simulink model "eVTOL_System"  (R2024b)
settings: Solver=FixedStepAuto  StartTime=0.0  StopTime=inf  RelTol=1e-3
undefined symbols (not defined in the file): airspeed, Battery, BCE12, BCE_Set_init, BMS_Controller_State, C, Cell10_P, Cell11_P, Cell12_P, Cell13_P, Cell14_P, Cell15_P, Cell16_P, Cell17_P, Cell18_P, Cell19_P, Cell1_N, Cell1_P, Cell20_P, Cell21_P, Cell22_P, Cell23_P, Cell24_P, Cell2_P, Cell3_P, Cell4_P, Cell5_P, Cell6_P, Cell7_P, Cell8_P, Cell9_P, Charging_State, CityMission, control, controlParams, ControlSampleTime, CriticalTiltAngle, currentFactor, CV_Gain, ddx, ddy, ddz, Device_01, Device_02, DiscIntNeverNeededParam, dx, dy, dz, Earth, env, F, F28379D_ADC_MaxCount, F28379D_ADC_Vmax, FixedWingMission, flightState, Foc_Ki_IxTcpu, Foc_Ki_S, Foc_Kp_I, Foc_Kp_S, fractalcoef ... (+68)
libraries: fl_lib x1115, nesl_utility x617, slrealtimeethercatlib x217, simulink x130, canmsglib x101, speedgoatlib_IO611_obsolete x91, slpidlib x49, mcbcontrolslib x44, slrealtimeutilitieslib x35, speedgoatlib_hdlCoder_IO3xx x31, dspstat3 x24, mcbpositiondecoderlib x12
(part 30 of 31)

== system eVTOL_System/Motor Drive/Controller2/Controller_MIL/F28379D Firmware/Controller Algorithm/FOC/Current Control/Control_System/Closed Loop Control/Subsystem/Current_Controllers/PI_Controller_Iq ==
  I_ref : Inport
  I_fb : Inport  Port=2
  EnablePWM : Inport  Port=3
  Kp_i : Inport  Port=4
  Ki_ixTcpu : Inport  Port=5
  Discrete PI Controller with anti-windup & reset : slpidlib/PID Controller  Controller=PI  Form=Parallel  TimeDomain=Discrete-time  UseExternalTs=off  SampleTime=-1  IntegratorMethod=Forward Euler  FilterMethod=Forward Euler  ControllerParametersSource=external  P=1  I=1  UseKiTs=on  D=0  UseExternalDerivativeSource=off  N=100  UseFilter=on  TunerSelectOption=Transfer Function Based (PID Tuner App)  InitialConditionSource=external  InitialConditionForIntegrator=0  InitialConditionForFilter=0  DifferentiatorICPrevScaledInput=0  ExternalReset=level  TrackingMode=off  Kt=1  LimitOutput=on  SatLimitsSource=internal  UpperSaturationLimit=1  LowerSaturationLimit=-1  LinearizeAsGain=on  AntiWindupMode=clamping  Kb=1  LimitIntegrator=off  UpperIntegratorSaturationLimit=inf  LowerIntegratorSaturationLimit=-inf  RndMeth=Simplest  POutMin=[]  POutMax=[]  IOutMin=[]  IOutMax=[]  DOutMin=[]  DOutMax=[]  NOutMin=[]  NOutMax=[]  SumOutMin=[]  SumOutMax=[]  SaturationOutDataTypeStr=Inherit: Inherit via back propagation  SaturationOutMin=[]  SaturationOutMax=[]  PParamMin=[]  PParamMax=[]  IParamMin=[]  IParamMax=[]  DParamMin=[]  DParamMax=[]  NParamMin=[]  NParamMax=[]  KbParamMin=[]  KbParamMax=[]  KtParamMin=[]  KtParamMax=[]  KbOutMin=[]  KbOutMax=[]  KtOutMin=[]  KtOutMax=[]  IntegratorOutMin=[]  IntegratorOutMax=[]  FilterOutMin=[]  FilterOutMax=[]  SumI1OutMin=[]  SumI1OutMax=[]  SumI2OutMin=[]  SumI2OutMax=[]  SumI3OutMin=[]  SumI3OutMax=[]  SumI4OutMin=[]  SumI4OutMax=[]  SumDOutMin=[]  SumDOutMax=[]  DifferentiatorOutMin=[]  DifferentiatorOutMax=[]  FilterDiffOutCoefMin=[]  FilterDiffOutCoefMax=[]  ReciprocalOutMin=[]  ReciprocalOutMax=[]  SumDenOutMin=[]  SumDenOutMax=[]  SumNumOutMin=[]  SumNumOutMax=[]  DivideOutMin=[]  DivideOutMax=[]  UdiffTsProdOutMin=[]  UdiffTsProdOutMax=[]  NTsProdOutMin=[]  NTsProdOutMax=[]  UintegralTsProdOutMin=[]  UintegralTsProdOutMax=[]  UngainTsProdOutMin=[]  UngainTsProdOutMax=[]  ClampingZeroOutDataTypeStr=Inherit: Inherit via back propagation  ClampingZeroOutMin=[]  ClampingZeroOutMax=[]  FilterDenConstantOutDataTypeStr=Inherit: Inherit via back propagation  FilterDenConstantOutMin=[]  FilterDenConstantOutMax=[]  PCopyOutDataTypeStr=Inherit: Inherit via back propagation  PCopyOutMin=[]  PCopyOutMax=[]  NCopyOutDataTypeStr=Inherit: Inherit via back propagation  NCopyOutMin=[]  NCopyOutMax=[]  IntegratorContinuousStateAttributes=''  IntegratorStateMustResolveToSignalObject=off  IntegratorRTWStateStorageClass=Auto  FilterContinuousStateAttributes=''  FilterStateMustResolveToSignalObject=off  FilterRTWStateStorageClass=Auto  ParallelPVariant=ExternalParameters  IdealPVariant=Disabled  IVariant=ExternalParameters  DVariant=Disabled  IntegratorVariant=Discrete  SatVariant=Enabled  AWVariant=DiscClampingParallel  PCopyVariant=Disabled  TRVariant=Disabled  FdbkBlocksVariant=Forward  IdealPFdbkVariant=Disabled  SatFdbkVariant=Disabled  DerivativeFilterVariant=Disabled  NVariant=Disabled  NCopyVariant=Disabled_SignalSpec  FilterICVariant=Disabled  IntegratorICVariant=ExternalICs  ExternalResetVariant=ExternalReset  TRSumVariant=Passthrough  SumFdbkVariant=Disabled  SumVariant=Sum_PI  TsampFilterVariant=InternalTs  TsampNgainVariant=Passthrough  TsampIntegralVariant=Disabled_SignalSpec  ExternalSaturationOutDataTypeStr=Inherit: Same as second input  DerivativeSourceVariant=Disabled  PreIntVariant=InternalPreInt
  Kp1 : Constant  Value=0  OutDataTypeStr=single  SampleTime=-1
  Logical Operator : Logic  Operator=NOT  IconShape=distinctive  AllPortsSameDT=off  OutDataTypeStr=boolean
  Sum : Sum  Inputs=|+-  OutDataTypeStr=Inherit: Same as first input
  V_ref : Outport  VectorParamsAs1DForOutWhenUnconnected=off
  wires:
  Discrete PI Controller with anti-windup & reset/1 -> V_ref/1
  I_fb/1 -> Sum/2
  I_ref/1 -> Sum/1
  Sum/1 -> Discrete PI Controller with anti-windup & reset/1
  Logical Operator/1 -> Discrete PI Controller with anti-windup & reset/4
  Kp1/1 -> Discrete PI Controller with anti-windup & reset/5
  EnablePWM/1 -> Logical Operator/1
  Kp_i/1 -> Discrete PI Controller with anti-windup & reset/2
  Ki_ixTcpu/1 -> Discrete PI Controller with anti-windup & reset/3

== system eVTOL_System/Motor Drive/Controller3/Controller_MIL/F28379D Firmware/Controller Algorithm/FOC/Current Control/Control_System/Closed Loop Control/Subsystem/Current_Controllers/PI_Controller_Id ==
  I_ref : Inport
  I_fb : Inport  Port=2
  EnablePWM : Inport  Port=3
  Kp_i : Inport  Port=4
  Ki_ixTcpu : Inport  Port=5
  Discrete PI Controller with anti-windup & reset : slpidlib/PID Controller  Controller=PI  Form=Parallel  TimeDomain=Discrete-time  UseExternalTs=off  SampleTime=-1  IntegratorMethod=Forward Euler  FilterMethod=Forward Euler  ControllerParametersSource=external  P=1  I=1  UseKiTs=on  D=0  UseExternalDerivativeSource=off  N=100  UseFilter=on  TunerSelectOption=Transfer Function Based (PID Tuner App)  InitialConditionSource=external  InitialConditionForIntegrator=0  InitialConditionForFilter=0  DifferentiatorICPrevScaledInput=0  ExternalReset=level  TrackingMode=off  Kt=1  LimitOutput=on  SatLimitsSource=internal  UpperSaturationLimit=1  LowerSaturationLimit=-1  LinearizeAsGain=on  AntiWindupMode=clamping  Kb=1  LimitIntegrator=off  UpperIntegratorSaturationLimit=inf  LowerIntegratorSaturationLimit=-inf  RndMeth=Simplest  POutMin=[]  POutMax=[]  IOutMin=[]  IOutMax=[]  DOutMin=[]  DOutMax=[]  NOutMin=[]  NOutMax=[]  SumOutMin=[]  SumOutMax=[]  SaturationOutDataTypeStr=Inherit: Inherit via back propagation  SaturationOutMin=[]  SaturationOutMax=[]  PParamMin=[]  PParamMax=[]  IParamMin=[]  IParamMax=[]  DParamMin=[]  DParamMax=[]  NParamMin=[]  NParamMax=[]  KbParamMin=[]  KbParamMax=[]  KtParamMin=[]  KtParamMax=[]  KbOutMin=[]  KbOutMax=[]  KtOutMin=[]  KtOutMax=[]  IntegratorOutMin=[]  IntegratorOutMax=[]  FilterOutMin=[]  FilterOutMax=[]  SumI1OutMin=[]  SumI1OutMax=[]  SumI2OutMin=[]  SumI2OutMax=[]  SumI3OutMin=[]  SumI3OutMax=[]  SumI4OutMin=[]  SumI4OutMax=[]  SumDOutMin=[]  SumDOutMax=[]  DifferentiatorOutMin=[]  DifferentiatorOutMax=[]  FilterDiffOutCoefMin=[]  FilterDiffOutCoefMax=[]  ReciprocalOutMin=[]  ReciprocalOutMax=[]  SumDenOutMin=[]  SumDenOutMax=[]  SumNumOutMin=[]  SumNumOutMax=[]  DivideOutMin=[]  DivideOutMax=[]  UdiffTsProdOutMin=[]  UdiffTsProdOutMax=[]  NTsProdOutMin=[]  NTsProdOutMax=[]  UintegralTsProdOutMin=[]  UintegralTsProdOutMax=[]  UngainTsProdOutMin=[]  UngainTsProdOutMax=[]  ClampingZeroOutDataTypeStr=Inherit: Inherit via back propagation  ClampingZeroOutMin=[]  ClampingZeroOutMax=[]  FilterDenConstantOutDataTypeStr=Inherit: Inherit via back propagation  FilterDenConstantOutMin=[]  FilterDenConstantOutMax=[]  PCopyOutDataTypeStr=Inherit: Inherit via back propagation  PCopyOutMin=[]  PCopyOutMax=[]  NCopyOutDataTypeStr=Inherit: Inherit via back propagation  NCopyOutMin=[]  NCopyOutMax=[]  IntegratorContinuousStateAttributes=''  IntegratorStateMustResolveToSignalObject=off  IntegratorRTWStateStorageClass=Auto  FilterContinuousStateAttributes=''  FilterStateMustResolveToSignalObject=off  FilterRTWStateStorageClass=Auto  ParallelPVariant=ExternalParameters  IdealPVariant=Disabled  IVariant=ExternalParameters  DVariant=Disabled  IntegratorVariant=Discrete  SatVariant=Enabled  AWVariant=DiscClampingParallel  PCopyVariant=Disabled  TRVariant=Disabled  FdbkBlocksVariant=Forward  IdealPFdbkVariant=Disabled  SatFdbkVariant=Disabled  DerivativeFilterVariant=Disabled  NVariant=Disabled  NCopyVariant=Disabled_SignalSpec  FilterICVariant=Disabled  IntegratorICVariant=ExternalICs  ExternalResetVariant=ExternalReset  TRSumVariant=Passthrough  SumFdbkVariant=Disabled  SumVariant=Sum_PI  TsampFilterVariant=InternalTs  TsampNgainVariant=Passthrough  TsampIntegralVariant=Disabled_SignalSpec  ExternalSaturationOutDataTypeStr=Inherit: Same as second input  DerivativeSourceVariant=Disabled  PreIntVariant=InternalPreInt
  Ki1 : Constant  Value=0  OutDataTypeStr=single  SampleTime=-1
  Logical Operator : Logic  Operator=NOT  IconShape=distinctive  AllPortsSameDT=off  OutDataTypeStr=boolean
  Sum : Sum  Inputs=|+-  OutDataTypeStr=Inherit: Same as first input
  V_ref : Outport  VectorParamsAs1DForOutWhenUnconnected=off
  wires:
  I_ref/1 -> Sum/1
  I_fb/1 -> Sum/2
  Discrete PI Controller with anti-windup & reset/1 -> V_ref/1
  Sum/1 -> Discrete PI Controller with anti-windup & reset/1
  Logical Operator/1 -> Discrete PI Controller with anti-windup & reset/4
  Ki1/1 -> Discrete PI Controller with anti-windup & reset/5
  EnablePWM/1 -> Logical Operator/1
  Kp_i/1 -> Discrete PI Controller with anti-windup & reset/2
  Ki_ixTcpu/1 -> Discrete PI Controller with anti-windup & reset/3

== system eVTOL_System/Motor Drive/Controller3/Controller_MIL/F28379D Firmware/Controller Algorithm/FOC/Current Control/Control_System/Closed Loop Control/Subsystem/Current_Controllers/PI_Controller_Iq ==
  I_ref : Inport
  I_fb : Inport  Port=2
  EnablePWM : Inport  Port=3
  Kp_i : Inport  Port=4
  Ki_ixTcpu : Inport  Port=5
  Discrete PI Controller with anti-windup & reset : slpidlib/PID Controller  Controller=PI  Form=Parallel  TimeDomain=Discrete-time  UseExternalTs=off  SampleTime=-1  IntegratorMethod=Forward Euler  FilterMethod=Forward Euler  ControllerParametersSource=external  P=1  I=1  UseKiTs=on  D=0  UseExternalDerivativeSource=off  N=100  UseFilter=on  TunerSelectOption=Transfer Function Based (PID Tuner App)  InitialConditionSource=external  InitialConditionForIntegrator=0  InitialConditionForFilter=0  DifferentiatorICPrevScaledInput=0  ExternalReset=level  TrackingMode=off  Kt=1  LimitOutput=on  SatLimitsSource=internal  UpperSaturationLimit=1  LowerSaturationLimit=-1  LinearizeAsGain=on  AntiWindupMode=clamping  Kb=1  LimitIntegrator=off  UpperIntegratorSaturationLimit=inf  LowerIntegratorSaturationLimit=-inf  RndMeth=Simplest  POutMin=[]  POutMax=[]  IOutMin=[]  IOutMax=[]  DOutMin=[]  DOutMax=[]  NOutMin=[]  NOutMax=[]  SumOutMin=[]  SumOutMax=[]  SaturationOutDataTypeStr=Inherit: Inherit via back propagation  SaturationOutMin=[]  SaturationOutMax=[]  PParamMin=[]  PParamMax=[]  IParamMin=[]  IParamMax=[]  DParamMin=[]  DParamMax=[]  NParamMin=[]  NParamMax=[]  KbParamMin=[]  KbParamMax=[]  KtParamMin=[]  KtParamMax=[]  KbOutMin=[]  KbOutMax=[]  KtOutMin=[]  KtOutMax=[]  IntegratorOutMin=[]  IntegratorOutMax=[]  FilterOutMin=[]  FilterOutMax=[]  SumI1OutMin=[]  SumI1OutMax=[]  SumI2OutMin=[]  SumI2OutMax=[]  SumI3OutMin=[]  SumI3OutMax=[]  SumI4OutMin=[]  SumI4OutMax=[]  SumDOutMin=[]  SumDOutMax=[]  DifferentiatorOutMin=[]  DifferentiatorOutMax=[]  FilterDiffOutCoefMin=[]  FilterDiffOutCoefMax=[]  ReciprocalOutMin=[]  ReciprocalOutMax=[]  SumDenOutMin=[]  SumDenOutMax=[]  SumNumOutMin=[]  SumNumOutMax=[]  DivideOutMin=[]  DivideOutMax=[]  UdiffTsProdOutMin=[]  UdiffTsProdOutMax=[]  NTsProdOutMin=[]  NTsProdOutMax=[]  UintegralTsProdOutMin=[]  UintegralTsProdOutMax=[]  UngainTsProdOutMin=[]  UngainTsProdOutMax=[]  ClampingZeroOutDataTypeStr=Inherit: Inherit via back propagation  ClampingZeroOutMin=[]  ClampingZeroOutMax=[]  FilterDenConstantOutDataTypeStr=Inherit: Inherit via back propagation  FilterDenConstantOutMin=[]  FilterDenConstantOutMax=[]  PCopyOutDataTypeStr=Inherit: Inherit via back propagation  PCopyOutMin=[]  PCopyOutMax=[]  NCopyOutDataTypeStr=Inherit: Inherit via back propagation  NCopyOutMin=[]  NCopyOutMax=[]  IntegratorContinuousStateAttributes=''  IntegratorStateMustResolveToSignalObject=off  IntegratorRTWStateStorageClass=Auto  FilterContinuousStateAttributes=''  FilterStateMustResolveToSignalObject=off  FilterRTWStateStorageClass=Auto  ParallelPVariant=ExternalParameters  IdealPVariant=Disabled  IVariant=ExternalParameters  DVariant=Disabled  IntegratorVariant=Discrete  SatVariant=Enabled  AWVariant=DiscClampingParallel  PCopyVariant=Disabled  TRVariant=Disabled  FdbkBlocksVariant=Forward  IdealPFdbkVariant=Disabled  SatFdbkVariant=Disabled  DerivativeFilterVariant=Disabled  NVariant=Disabled  NCopyVariant=Disabled_SignalSpec  FilterICVariant=Disabled  IntegratorICVariant=ExternalICs  ExternalResetVariant=ExternalReset  TRSumVariant=Passthrough  SumFdbkVariant=Disabled  SumVariant=Sum_PI  TsampFilterVariant=InternalTs  TsampNgainVariant=Passthrough  TsampIntegralVariant=Disabled_SignalSpec  ExternalSaturationOutDataTypeStr=Inherit: Same as second input  DerivativeSourceVariant=Disabled  PreIntVariant=InternalPreInt
  Kp1 : Constant  Value=0  OutDataTypeStr=single  SampleTime=-1
  Logical Operator : Logic  Operator=NOT  IconShape=distinctive  AllPortsSameDT=off  OutDataTypeStr=boolean
  Sum : Sum  Inputs=|+-  OutDataTypeStr=Inherit: Same as first input
  V_ref : Outport  VectorParamsAs1DForOutWhenUnconnected=off
  wires:
  Discrete PI Controller with anti-windup & reset/1 -> V_ref/1
  I_fb/1 -> Sum/2
  I_ref/1 -> Sum/1
  Sum/1 -> Discrete PI Controller with anti-windup & reset/1
  Logical Operator/1 -> Discrete PI Controller with anti-windup & reset/4
  Kp1/1 -> Discrete PI Controller with anti-windup & reset/5
  EnablePWM/1 -> Logical Operator/1
  Kp_i/1 -> Discrete PI Controller with anti-windup & reset/2
  Ki_ixTcpu/1 -> Discrete PI Controller with anti-windup & reset/3

== matlab function eVTOL_System/Flight Controller/Autopilot/Fixed Wing Controller/Fixed Wing Controller Simulation/Attitude Controller/Pitch Roll Controller/Turn Coordinator/MATLAB Function ==
  data: rollSP input; rSP output; pitchSP input; airSpeed input
function rSP = fcn(rollSP, pitchSP, airSpeed)
    yawRateSP = tan(rollSP)*9.81/airSpeed;
    rSP = yawRateSP*cos(pitchSP)*cos(rollSP);
end

== stateflow chart eVTOL_System/Flight Controller/Guidance Test Bench/ControlType/Guidance Testbench/Guidance Logic/Guidance Stateflow/Guidance Mode Selector ==
  settings: updateMethod=DISCRETE  sampleTime=UAVSampleTime*4
  state GuidanceLogic
    state FIXED_WING_WAYPOINT
      en:
      controlMode.airspeedAltitude = 1;
      controlMode.attitude = 1;
      controlMode.lateralGuidance = 1;
      state WAYPOINT
    state FIXED_WING_ENTRY
      state Stabilize
        en:
        FlightMode=flightState.FixedWing;
        controlMode.attitude = 1;
        controlMode.airspeedAltitude = 0;
        controlMode.lateralGuidance = 0;
        %Transition once done.
        FixedWingSP.yaw = 0;
        FixedWingSP.pitch = 0;
        FixedWingSP.roll = 0;
        FixedWingSP.airspeed=14;
        Status= uint8(0);
      state FIXEDWINGFLIGHT
        en:
        % Control mode
        controlMode.airspeedAltitude = 1;
        controlMode.attitude = 1;
        controlMode.lateralGuidance = 1;
        % Setpoint init
        aacSP.L1 = 25;
        aacSP.airspeed = 14;
        aacSP.altitude = 0;
        aacSP.course=0;
      (default) -> Stabilize
      Stabilize -> FIXEDWINGFLIGHT : after(3,sec)
    state Start
      en:
      %Set Flight mode to hover
      FlightMode=PresetMode;
      %Set default settings
      % Control mode
      controlMode.airspeedAltitude = 0;
      controlMode.attitude = 0;
      controlMode.lateralGuidance = 0;
      controlMode.TransitionCondition = 0;
      % Setpoint init
      FixedWingSP.yaw = 0;
      FixedWingSP.pitch = 0;
      FixedWingSP.roll = 0;
      FixedWingSP.airspeed=14;
      aacSP.L1 = 25;
      aacSP.airspeed = 14;
      aacSP.altitude = 0;
      aacSP.course=0;
      InnerLoopCmds.YawCmd=0;
    state FIXED_WING_ORBIT
      en:
      controlMode.airspeedAltitude = 1;
      controlMode.attitude = 1;
      controlMode.lateralGuidance = 1;
      state ORBIT
    state HOVER_ENTRY
      en:
      FlightMode=flightState.Hover;
      controlMode.inTransition=0;
    state Takeoff
    state WP
    state Orbit
    state PreTransition
      en:
      FlightMode=flightState.FixedWing;
      controlMode.airspeedAltitude = 1;
      controlMode.attitude = 1;
      controlMode.lateralGuidance = 1;
      % Setpoint init
      aacSP.L1 = 25;
      aacSP.airspeed = 14;
      aacSP.altitude = altitudeHold;
      aacSP.course=courseHold;
    state BackTransition
      state BackTransition
    state ForwardTransition
    state FWCOMPLETE
      Status=uint8(1);
      controlMode.TransitionCondition=uint8(1);
    note: [(mode==4)]
    state Land
      state Descend
      state WingsLevel
      state ToLand
      (default) -> ToLand
      WingsLevel -> Descend : [isLevel(States)]
      ToLand -> WingsLevel : [(norm(Pose(1:2)-ToWP.position(1:2)) <= 5)]
    (default) -> Start
    Start -> (junction 5)
    FIXEDWINGFLIGHT -> WAYPOINT [order 2] : [(mode==2)]
        | {Status=uint8(0);}
    FIXEDWINGFLIGHT -> ORBIT [order 1] : [(mode==3)]
        | {Status= uint8(0);}
    (junction 262) -> FIXED_WING_ENTRY
    (junction 5) -> FIXED_WING_ORBIT [order 6] : [(mode==3)&&(FlightMode==flightState.FixedWing)]
        | {Status=uint8(0);}
    (junction 5) -> (junction 262) [order 3] : [(FlightMode==flightState.Transition)]
        | {controlMode.inTransition=0;}
    (junction 255) -> HOVER_ENTRY
    (junction 5) -> (junction 255) [order 4] : [(FlightMode==flightState.BackTransition)]
        | {controlMode.inTransition=0;}
    HOVER_ENTRY -> (junction 12)
    (junction 257) -> FIXED_WING_WAYPOINT
    Takeoff -> WP : [Pose(3) <= ToWP.position(3)]{Status = uint8(1);}
    GuidanceLogic -> (junction 5) : [(hasChanged(mode))]
    (junction 5) -> Takeoff [order 5] : [(mode == 1)&&(FlightMode==flightState.Hover)]
        | {controlMode.inTransition=0;}
    (junction 5) -> (junction 257) [order 2] : [(mode==2)&&(FlightMode==flightState.FixedWing)]
        | {Status=uint8(0);}
    (junction 5) -> (junction 260) [order 1] : [(mode==6)&&(FlightMode==flightState.FixedWing)]
        | {courseHold=States.course;
        | altitudeHold=-States.Xe(3); }
    (junction 5) -> (junction 12) [order 7] : [FlightMode==flightState.Hover]
        | {controlMode.inTransition=0;}
    (junction 260) -> PreTransition
    (junction 12) -> WP [order 1] : [(mode==2)]
    (junction 12) -> (junction 17) [order 2]
    (junction 17) -> Orbit [order 1] : [(mode==3)]
    (junction 17) -> (junction 22) [order 2]
    PreTransition -> GuidanceLogic.BackTransition : after(5,sec)
        | {FlightMode=flightState.BackTransition;
        | controlMode.inTransition=1; }
    (junction 22) -> ForwardTransition [order 1] : [(mode==6)]
        | {FlightMode=flightState.Transition;
        | controlMode.inTransition=1;
        | controlMode.TransitionCondition=uint8(0);
        |
        | }
    (junction 22) -> Land [order 2]
    ForwardTransition -> FWCOMPLETE : [transitionConditionMet(States,Vt)]
    Land -> GuidanceLogic : [abs(Pose(3)-zGround)<=0.1]{Status = uint8(2);}
  (default) -> GuidanceLogic
  data: sf_internal_action_state_placeholder_data local double size=1 =0; sf_internal_action_state_placeholder_data local double size=1 =0; sf_internal_action_state_placeholder_data local double size=1 =0; sf_internal_action_state_placeholder_data local double size=1 =0; sf_internal_action_state_placeholder_data local double size=1 =0; sf_internal_action_state_placeholder_data local double size=1 =0; sf_internal_action_state_placeholder_data local double size=1 =0; sf_internal_action_state_placeholder_data local double size=1 =0; sf_internal_action_state_placeholder_data local double size=1 =0; sf_internal_action_state_placeholder_data local double size=1 =0; AttitudeState function_input Bus: GuidanceStates; valid function_output; TransitionSt function_input Bus: GuidanceStates; valid function_output; Vtransition function_input; mode input; ToWP input Bus: doubleUavPathManager; Status output uint8; FromWP input Bus: doubleUavPathManager; Pose input; GdncMode output Enum: GdncModeType; States input; aacSP output Bus: AAC; FixedWingSP output Bus: FixedWingCommandBus; controlMode output Bus: controlMode; FlightMode output; PresetMode input; courseHold local; altitudeHold local; Vt parameter double; InnerLoopCmds output Bus: innerLoopCmdsBus; zGround parameter
  function valid=isLevel(AttitudeState):
    | function valid=isLevel(AttitudeState)
    | %wingsLevel
    | if(norm(AttitudeState.Euler)<1e-1)&&(norm(AttitudeState.pqr)<1e-1)
    |    valid=true;
    | else
    |     valid=false;
    | end
    | 
    | end
  function valid=transitionConditionMet(TransitionSt,Vtransition):
    | function valid=transitionConditionMet(TransitionSt,Vtransition)
    | %wingsLevel
    | if(States.Tilt>=1.57)&&(vecnorm(States.Ve)>Vt)
    |    valid=true;
    | else
    |     valid=false;
    | end
    | end

== matlab function eVTOL_System/Flight Controller/Guidance Test Bench/ControlType/Guidance Testbench/Guidance Logic/Guidance Stateflow/Guidance Mode Selector/GuidanceLogic.Land.ToLand/MATLAB Function ==
  data: FromWP input Bus: doubleUavPathManager size=1; wps output; ToWP input Bus: doubleUavPathManager size=1
function wps = getLandingWaypoint(FromWP, ToWP)

persistent outWPS

if isempty(outWPS)
    outWPS = double(zeros(2,4));
end

outWPS(1,:) = [FromWP.position' FromWP.params(4)];
outWPS(2,:) = [ToWP.position(1:2)' FromWP.position(3) ToWP.params(4)];

wps = outWPS;

== stateflow chart eVTOL_System/Battery System/BMS/MIL/Controller/Balancing Logic/Balancing ==
  settings: updateMethod=DISCRETE
  state BalancingOFF
    en:
    Bal_Cmd(:,:) = false;
    en,du:
    MaxCellVolt = max(CellVoltages);
    MinCellVolt = min(CellVoltages);
    DeltaCellVolt = MaxCellVolt - MinCellVolt;
  state BalancingON
    en, du:
    MaxCellVolt = max(CellVoltages);
    MinCellVolt = min(CellVoltages);
    DeltaCellVolt = MaxCellVolt - MinCellVolt;
    state BalActive
      en, du:
      Bal_Cmd = ((CellVoltages - MinCellVolt) > TargetDeltaV)';
      flgBalCompl = all(~Bal_Cmd);
    state BalNotActive
    (default) -> BalActive
    BalNotActive -> BalActive [order 1] : [after(BalNotActWait,sec) && ...
        | DeltaCellVolt > TargetDeltaV]
    BalActive -> BalNotActive : [flgBalCompl]
  note: "Copyright 2018 - 2019 The MathWorks, Inc."
  (default) -> BalancingOFF : {flgBalCompl = true;}
  BalancingOFF -> BalancingON : [flgEnBalancing && ...
      | BMS_State ~= BMS_Controller_State.BMS_Driving && ...
      | BMS_State ~= BMS_Controller_State.BMS_Fault && ...
      | after(BalOffWait,sec) && ...
      | DeltaCellVolt > TargetDeltaV]
  BalancingON -> BalancingOFF : [BMS_State == BMS_Controller_State.BMS_Driving]
  BalNotActive -> BalancingOFF [order 2] : [after(BalOnWait,sec)]
  data: BMS_State input Enum: BMS_Controller_State; CellVoltages input single; Bal_Cmd output boolean size=[1,Ns_Module*NumModules] =boolean(zeros(1, Ns_Module*NumModules)); flgBalCompl local; BalNotActWait local =int16(10); BalOffWait local =int16(5); BalOnWait local =int16(20); flgEnBalancing local =boolean(1); DeltaCellVolt local single =single(0); MaxCellVolt local =single(4); MinCellVolt local =single(3); TargetDeltaV local =single(0.1)

== matlab function eVTOL_System/Flight Controller/Guidance Test Bench/ControlType/Guidance Testbench/Guidance Logic/Guidance Stateflow/Guidance Mode Selector/GuidanceLogic.Land.WingsLevel/MATLAB Function ==
  data: FromWP input Bus: doubleUavPathManager size=1; outWPS output; ToWP input Bus: doubleUavPathManager size=1
function outWPS = getDestinationWaypoint(FromWP, ToWP)

outWPS=zeros(1,3);

outWPS(1,:) = [ToWP.position(1:2)' FromWP.position(3)];

end

== matlab function eVTOL_System/Flight Controller/Guidance Test Bench/ControlType/Guidance Testbench/Guidance Logic/Guidance Stateflow/Guidance Mode Selector/GuidanceLogic.WP/MATLAB Function ==
  data: FromWP input Bus: doubleUavPathManager size=1; wps output; ToWP input Bus: doubleUavPathManager size=1
function wps = getWaypointMission(FromWP, ToWP)

persistent outWPS

if isempty(outWPS)
    outWPS = double(zeros(2,4));
end

outWPS(1,:) = [FromWP.position' FromWP.params(4)];
outWPS(2,:) = [ToWP.position' ToWP.params(4)];

wps = outWPS;

== matlab function eVTOL_System/Flight Controller/Guidance Test Bench/ControlType/Guidance Testbench/Guidance Logic/Guidance Stateflow/Guidance Mode Selector/GuidanceLogic.FIXED_WING_WAYPOINT.WAYPOINT/MATLAB Function ==
  data: toWP input; wps output; fromWP input; alt output
function [wps, alt]= fcn(toWP, fromWP)
    wps = zeros(2,3); %#ok<PREALL> 
    wps = [fromWP'; toWP'];
    alt = -toWP(3);
end

== matlab function eVTOL_System/Battery System/Battery/Battery Pack/100-Cell/Trigger_Faults/Short-Circuit_Faults ==
  data: CellNumber input; ShortCircuit output size=100; Enable input; Reset input; Feedback input size=100
function ShortCircuit = fcn(CellNumber,Enable,Reset,Feedback)

if Reset
    Feedback = zeros(100,1);        
end

for i=1:100
    if Enable && CellNumber == i
        Feedback(i) = true;
    end    
end

ShortCircuit = Feedback;

end

== matlab function eVTOL_System/Flight Controller/Autopilot/Fixed Wing Controller/Fixed Wing Controller Simulation/Subsystem2/MATLAB Function ==
  data: phi input; y output; theta input
function y = fcn(phi,theta)

y=zeros(3,3);
y=[1 sin(phi)*tan(theta) cos(phi)*tan(theta); 0 cos(phi) -sin(phi); 0 sin(phi)/cos(theta) cos(phi)/cos(theta)];
end

== stateflow chart eVTOL_System/Flight Controller/Guidance Test Bench/ControlType/Manual Control/Command Interface/Basic Control  Switching ==
  state STATE_MACHINE
    state DEFAULT
      en:
      controlMode.lateralGuidance=1;
      controlMode.airspeedAltitude=1;
      controlMode.attitude=1;
      controlMode.manual=0;
      controlMode.armed=0;
      controlMode.inTransition=0;
    state TRANSITION
      controlMode.lateralGuidance=1;
      controlMode.airspeedAltitude=1;
      controlMode.attitude=1;
      controlMode.manual=0;
      controlMode.armed=0;
      controlMode.inTransition=1;
      controlMode.TransitionCondition=0;
    (default) -> DEFAULT
    STATE_MACHINE -> DEFAULT [order 2] : [hasChanged(FlightMode)]
    STATE_MACHINE -> TRANSITION [order 1] : [hasChanged(FlightMode)&&((FlightMode==flightState.Transition)||(FlightMode==flightState.BackTransition))]
    TRANSITION -> STATE_MACHINE [order 2] : [backConditioMet(States)&&(FlightMode==flightState.BackTransition)]
        | {controlMode.TransitionCondition=1;
        | controlMode.inTransition=0;}
    TRANSITION -> STATE_MACHINE [order 1] : [transitionConditionMet(States,Vt)&&(FlightMode==flightState.Transition)]
        | {controlMode.TransitionCondition=1;
        | controlMode.inTransition=0;}
  data: TransitionStates function_input Bus: GuidanceStates; valid function_output; Vtransition function_input; TransitionStates function_input Bus: GuidanceStates; valid function_output; controlMode output Bus: controlMode; FlightMode input; States input; Vt parameter double
  function valid=transitionConditionMet(TransitionStates,Vtransition):
    | function valid=transitionConditionMet(TransitionStates,Vtransition)
    | %wingsLevel
    | if((States.Tilt>=1.57)&&(vecnorm(States.Ve)>Vt))
    |    valid=true;
    | else
    |     valid=false;
    | end
    | end
  function valid=backConditioMet(TransitionStates):
    | function valid=backConditioMet(TransitionStates)
    | %wingsLevel
    | if(vecnorm(States.Ve)<1e-1)
    |    valid=true;
    | else
    |     valid=false;
    | end
    | end

== matlab function eVTOL_System/Battery System/Battery/HW Interface/BCE - HIL/Battery Cell Emulator/BCE Write /Subsystem/BCE Write /MATLAB Function ==
  data: nodeNbr input; enable output; simTime input; Ts input
function enable = fcn(nodeNbr, simTime, Ts)
    % nodes 1, 21, 41, ... will send in the first 50 of each 1000 time steps
    % nodes 2, 22, 42, ... will send in the 51 to 100 of each 1000 time steps
    % and so on
    count = mod(simTime / Ts, 1000);
    sendWindow = mod(nodeNbr - 1, 20) * 50;
    enable = count > sendWindow && count < (sendWindow + 50);
end

== matlab function eVTOL_System/Battery System/Battery/HW Interface/BCE - HIL/Battery Cell Emulator/BCE Write 1/Subsystem/BCE Write /MATLAB Function ==
  data: nodeNbr input; enable output; simTime input; Ts input
function enable = fcn(nodeNbr, simTime, Ts)
    % nodes 1, 21, 41, ... will send in the first 50 of each 1000 time steps
    % nodes 2, 22, 42, ... will send in the 51 to 100 of each 1000 time steps
    % and so on
    count = mod(simTime / Ts, 1000);
    sendWindow = mod(nodeNbr - 1, 20) * 50;
    enable = count > sendWindow && count < (sendWindow + 50);
end

== matlab function eVTOL_System/Battery System/Battery/Override/MATLAB Function ==
  data: CellNumber input; VValue input; TValue input; InputVal input; VEnable input; Output1 output; Output2 output; Output3 output size=1; Output4 output size=1; Output5 output size=1; Output6 output size=1; TArrayFb output; TEnable input; UpdateVValue input; UpdateTValue input; Broken_wire input; Reset input; Wire_reset input; TArray input size=[1,100]; VArray input size=[1, 100]; VArrayFb output; flagFb output; BrokenWireFb output; flag input size=1; BrokenWires input size=[100,1]
function [Output1,Output2,Output3,Output4,Output5,Output6,TArrayFb,VArrayFb,flagFb,BrokenWireFb] = fcn(CellNumber, VValue, TValue, InputVal, VEnable, TEnable, UpdateVValue,UpdateTValue, Broken_wire, Reset,Wire_reset, TArray, VArray, flag, BrokenWires)
   
    if Reset
        VArray = zeros(1,100);
        TArray = zeros(1,100);        
    end

    if Wire_reset
        BrokenWires = zeros(100,1);
        flag = 0;
    end    

    if UpdateVValue ~= 1 
        UpdateVValue = 0;
    end

    if UpdateTValue ~= 1 
        UpdateTValue = 0;
    end

    if UpdateVValue && VEnable
        VArray(CellNumber) = VValue;        
    end
        
    if UpdateTValue && TEnable
        TArray(CellNumber) = TValue;
    end
    
    if VEnable
        for i=1:length(VArray)
            if VArray(i) ~= 0
                InputVal(i) = VArray(i);
            end
        end
    end
            
    if TEnable
        for j=101:(length(TArray)+100)        
            if TArray(j-100) ~= 0
                InputVal(j) = TArray(j-100);
            end
        end
    end    

    if Broken_wire
        BrokenWires(CellNumber) = 1;        
        for i=1:100
            if BrokenWires(i)
                InputVal(i) = 0;
            end
        end        
        flag = 1;
    end

    if flag
        for i=1:100
            if BrokenWires(i)
                InputVal(i) = 0;
            end
        end 
    end    
    
    Output1 = InputVal(1:100);
    Output2 = InputVal(101:200);
    Output3 = InputVal(201);
    Output4 = InputVal(202);
    Output5 = InputVal(203);
    Output6 = InputVal(204);
   
    VArrayFb = VArray;
    TArrayFb = TArray;
    BrokenWireFb = BrokenWires;
    flagFb = flag;
end

== matlab function eVTOL_System/Battery System/Instrumentation/Instrumented Signals/100-Cell/Display Cell Values ==
  data: CellNumber input; CellVoltages input; displayV output; CellTemperatures input; displayT output; displaySOC output; displayI output; CellSOC input; CellI input
function [displayV,displayT,displaySOC,displayI] = fcn(CellNumber, CellVoltages,CellTemperatures,CellSOC,CellI)
    displayV = 0;
    displayT = 0;
    displaySOC = 0;
    displayI = 0;

    for i=1:100
        if CellNumber == i
            displayV = CellVoltages(CellNumber);
            displayT = CellTemperatures(CellNumber);
            displaySOC = CellSOC(CellNumber);
            displayI = CellI(CellNumber);
        end
    end

end

== matlab function eVTOL_System/Dynamics/Ground Truth Bus/MATLAB Function1 ==
  data: vxyz input; course output; gndSpeed output
function [course, gndSpeed] = fcn(vxyz)

vx = vxyz(1);
vy = vxyz(2);
course = atan2(vy, vx);
gndSpeed = norm([vx vy 0]);

== matlab function eVTOL_System/Flight Controller/Autopilot/Fixed Wing Controller/Fixed Wing Controller Simulation/Lateral Guidance Logic/MATLAB Function ==
  data: courseSP input; lacc output; course input; rollSP output; groundSpeed input; L1 input
function [lacc, rollSP] = fcn(courseSP, course, groundSpeed, L1)
eta = courseSP - course;

% wrap -pi to pi
eta = mod(eta, 2*pi);
if eta>pi
    eta = eta - 2*pi;
end

% cap eta to -pi/2 to pi/2
eta = min(eta, pi/2);
eta = max(eta, -pi/2);

lacc = 2*(groundSpeed^2)/L1*sin(eta);

rollSP = atan(lacc/9.81);

== matlab function eVTOL_System/Dynamics/Variant Subsystem/No Sensors/MATLAB Function ==
  data: euler input; ypr output
function ypr = fcn(euler)

ypr = [euler(3),euler(2),euler(1)];
end

== stateflow chart eVTOL_System/Battery System/BMS/HIL/Controller_76Cells/BMS State Machine/State_Machine ==
  settings: updateMethod=DISCRETE  sampleTime=ts_controller
  state MainStateMachine [parallel]
    settings: executionOrder=1
    state Standby
      en:
      BMS_State = ...
      BMS_Controller_State.BMS_Idle;
    state Charging
      en:
      BMS_State = BMS_Controller_State.BMS_Charging;
      state Init_Mode
        en:
        ChargeModeReq = Charging_State.Init;
        ChargeCurrentReq = noCurrent;
      state CC_Mode
        en:
        ChargeModeReq = Charging_State.CC;
        du:
        ChargeCurrentReq = min(I_cc,ChargeCurrentLimit);
      state CV_Mode
        en:
        ChargeModeReq = Charging_State.CV;
        du:
        ChargeCurrentReq = ChargeCurrentReq - CV_Gain*(MaxCellVolt - MaxCellVoltThrsld);
        ChargeCurrentReq = min(ChargeCurrentReq, ChargeCurrentLimit);
      (default) -> Init_Mode
      CV_Mode -> Init_Mode : [State_Request ~= SRE.Charging || ...
          | ChargeCurrentReq <= (I_cc/currentFactor)]
      CC_Mode -> Init_Mode [order 1] : [State_Request ~= ...
          | SRE.Charging]
      Init_Mode -> CC_Mode : [State_Request == SRE.Charging && ...
          | MaxCellVolt < voltThreshold]
      CC_Mode -> CV_Mode [order 2] : [MaxCellVolt>=...
          | MaxCellVoltThrsld]
    state Driving
      en:
      BMS_State = ...
      BMS_Controller_State.BMS_Driving;
    state Fault
      en,du:
      BMS_State = ...
      BMS_Controller_State.BMS_Fault;
    (default) -> Standby
    Standby -> Fault [order 1] : [FaultPresent == true]
    Standby -> Charging [order 2] : [State_Request == SRE.Charging]
    (junction 699) -> Standby : [after(3,sec)]
    Charging -> Standby [order 3] : [State_Request ~= SRE.Charging]
    Standby -> Driving [order 3] : [State_Request == SRE.Flying]
    Driving -> Standby [order 3] : [State_Request ~= SRE.Flying]
    Driving -> Charging [order 2] : [State_Request == SRE.Charging]
    Charging -> Driving [order 2] : [State_Request == SRE.Flying]
    Fault -> (junction 699) : [[FaultPresent == false && Fault_Reset_Enable]]
    Driving -> Fault [order 1] : [FaultPresent]
    Charging -> Fault [order 1] : [FaultPresent]{ChargeCurrentReq = single(0);}
  state FaultMonitoring [parallel]
    settings: executionOrder=2
    state MonitorCellVoltage [parallel]
      settings: executionOrder=1
      state OverVoltageFault
        en:
        FaultPresent = true;
        Fault_out.OverVolt = true;
        du:
        MaxCellVolt = max(Cell_Voltages);
      state NoCellVoltFault
        en,du:
        MaxCellVolt = max(Cell_Voltages);
        MinCellVolt = min(Cell_Voltages);
      state UnderVoltageFault
        en:
        FaultPresent = true;
        Fault_out.UnderVolt = true;
        du:
        MinCellVolt = min(Cell_Voltages);
      OverVoltageFault -> (junction 687) : [MaxCellVolt < OverCellVoltageLimit && ...
          | Fault_Reset_Enable ...
          | ]{Fault_out.OverVolt=false; ...
          | FaultPresent = false;}
      (junction 695) -> OverVoltageFault : [after(100,msec)]
      NoCellVoltFault -> (junction 695) [order 1] : [MaxCellVolt >= ...
          | OverCellVoltageLimit]
      (junction 687) -> NoCellVoltFault : [after(3,sec)]
      (default) -> NoCellVoltFault : {FaultPresent = false;
          | Fault_out.OverVolt = false;
          | Fault_out.UnderVolt = false;}
      NoCellVoltFault -> (junction 697) [order 2] : [MinCellVolt <=...
          |  UnderCellVoltageLimit]
      (junction 685) -> NoCellVoltFault : [after(3,sec)]
      (junction 697) -> UnderVoltageFault : [after(100,msec)]
      UnderVoltageFault -> (junction 685) : [MinCellVolt > UnderCellVoltageLimit && ...
          | Fault_Reset_Enable] ...
          | {Fault_out.UnderVolt=false; ...
          | FaultPresent = false;}
    state MonitorCurrLim [parallel]
      settings: executionOrder=3
      state NoCurrLimFault
        en:
        FaultPresent = false;
        Fault_out.OverCurrent = false;
      state OverCurrentFault
        en:
        FaultPresent = true;
        Fault_out.OverCurrent=true;
      (default) -> NoCurrLimFault : {FaultPresent = false;
          | Fault_out.OverCurrent=false;}
      (junction 678) -> NoCurrLimFault : [after(3,sec)]
      NoCurrLimFault -> (junction 675) : [((DischargeCurrentLimit - Pack_Current) > single(0.2) && ...
          | BMS_State == BMS_Controller_State.BMS_Driving) || ...
          | ((Pack_Current - ChargeCurrentLimit) > single(0.2) && ...
          | BMS_State == BMS_Controller_State.BMS_Charging)]
      OverCurrentFault -> (junction 678) : [(Pack_Current >= DischargeCurrentLimit || ...
          |  Pack_Current <= ChargeCurrentLimit) && ...
          | Fault_Reset_Enable]
      (junction 675) -> OverCurrentFault : [after(100,msec)]
    state MonitorCellTemp [parallel]
      settings: executionOrder=2
      state HighTemperatureFault
        en:
        FaultPresent = true;
        Fault_out.HighTemp = true;
        du:
        MaxCellTemp = max(Cell_Temperatures);
      state NoCellTempFault
        en,du:
        MaxCellTemp = max(Cell_Temperatures);
        MinCellTemp = min(Cell_Temperatures);
      state LowTemperatureFault
        en:
        FaultPresent = true;
        Fault_out.LowTemp = true;
        du:
        MinCellTemp = min(Cell_Temperatures);
      HighTemperatureFault -> (junction 680) : [MaxCellTemp < HighTempLimit && ...
          | Fault_Reset_Enable] ...
          | {Fault_out.HighTemp=false; FaultPresent = false;}
      (junction 689) -> HighTemperatureFault : [after(100,msec)]
      (junction 680) -> NoCellTempFault : [after(3,sec)]
      NoCellTempFault -> (junction 689) [order 1] : [MaxCellTemp >= HighTempLimit]
      (default) -> NoCellTempFault : {FaultPresent = false;
          | Fault_out.HighTemp = false;
          | Fault_out.LowTemp = false;}
      (junction 682) -> NoCellTempFault : [after(3,sec)]
      NoCellTempFault -> (junction 691) [order 2] : [MinCellTemp <= LowTempLimit]
      LowTemperatureFault -> (junction 682) : [MinCellTemp > LowTempLimit && ...
          | Fault_Reset_Enable ] ...
          | {Fault_out.LowTemp=false; FaultPresent = false;}
      (junction 691) -> LowTemperatureFault : [after(100,msec)]
  data: DischargeCurrentLimit input single; ChargeCurrentLimit input single; State_Request input; Cell_Voltages input single; Pack_Voltage input single; Cell_Temperatures input single; Pack_Current input single; ChargeCurrentReq output; I_cc parameter; MaxCellVoltThrsld parameter; FaultPresent local; MaxCellTemp local; OverCellVoltageLimit parameter; UnderCellVoltageLimit parameter; MinCellTemp local; CV_Gain parameter; MonitorCurrLimMode local Enum: MonitorCurrLimModeType; MonitorCellVoltageMode local Enum: MonitorCellVoltageModeType; MonitorCellTempMode local Enum: MonitorCellTempModeType; Fault_out output Bus: Faults; voltThreshold parameter single; currentFactor parameter single; noCurrent parameter single; Fault_Reset_Enable input boolean; ChargeModeReq output Enum: Charging_State =Charging_State.Init; BMS_State output Enum: BMS_Controller_State =BMS_Controller_State.BMS_Idle; MaxCellVolt local; MinCellVolt local; HighTempLimit local =single(323.15); LowTempLimit local =single(278.15)

== stateflow chart eVTOL_System/Battery System/BMS/HIL/Controller_76Cells/Balancing Logic/Balancing ==
  settings: updateMethod=DISCRETE
  state BalancingOFF
    en:
    Bal_Cmd1(:,:) = false;
    en,du:
    MaxCellVolt = max(CellVoltages);
    MinCellVolt = min(CellVoltages);
    DeltaCellVolt = MaxCellVolt - MinCellVolt;
  state BalancingON
    en, du:
    MaxCellVolt = max(CellVoltages);
    MinCellVolt = min(CellVoltages);
    DeltaCellVolt = MaxCellVolt - MinCellVolt;
    state BalActive
      en, du:
      Bal_Cmd1 = ((CellVoltages - MinCellVolt) > TargetDeltaV)';
      flgBalCompl = all(~Bal_Cmd1);
    state BalNotActive
    (default) -> BalActive
    BalNotActive -> BalActive [order 1] : [after(BalNotActWait,sec) && ...
        | DeltaCellVolt > TargetDeltaV]
    BalActive -> BalNotActive : [flgBalCompl]
  note: "Copyright 2018 - 2019 The MathWorks, Inc."
  (default) -> BalancingOFF : {flgBalCompl = true;}
  BalancingOFF -> BalancingON : [flgEnBalancing && ...
      | BMS_State ~= BMS_Controller_State.BMS_Driving && ...
      | BMS_State ~= BMS_Controller_State.BMS_Fault && ...
      | after(BalOffWait,sec) && ...
      | DeltaCellVolt > TargetDeltaV]
  BalancingON -> BalancingOFF : [BMS_State == BMS_Controller_State.BMS_Driving]
  BalNotActive -> BalancingOFF [order 2] : [after(BalOnWait,sec)]
  data: BMS_State input Enum: BMS_Controller_State; CellVoltages input single; Bal_Cmd1 output boolean size=[1,76] =boolean(zeros(1, 76)); flgBalCompl local; BalNotActWait local =int16(10); BalOffWait local =int16(5); BalOnWait local =int16(20); flgEnBalancing local =boolean(1); DeltaCellVolt local single =single(0); MaxCellVolt local =single(4); MinCellVolt local =single(3); TargetDeltaV local =single(0.1)

== matlab function eVTOL_System/Flight Controller/Autopilot/Fixed Wing Controller/Fixed Wing Controller Tuning/Subsystem2/MATLAB Function ==
  data: phi input; y output; theta input
function y = fcn(phi,theta)

y=zeros(3,3);
y=[1 sin(phi)*tan(theta) cos(phi)*tan(theta); 0 cos(phi) -sin(phi); 0 sin(phi)/cos(theta) cos(phi)/cos(theta)];
end

== matlab function eVTOL_System/Dynamics/Force and Moments/Aerodynamic Drag/calcDragVector ==
  data: airVel input; dragVec output; dragCoeff input
function dragVec = fcn(airVel, dragCoeff)

dragVec = dragCoeff * norm(airVel) * airVel;

end

== matlab function eVTOL_System/Flight Controller/Autopilot/Fixed Wing Controller/Fixed Wing Controller Tuning/Lateral Guidance Logic/MATLAB Function ==
  data: courseSP input; lacc output; course input; rollSP output; groundSpeed input; L1 input
function [lacc, rollSP] = fcn(courseSP, course, groundSpeed, L1)
eta = courseSP - course;

% wrap -pi to pi
eta = mod(eta, 2*pi);
if eta>pi
    eta = eta - 2*pi;
end

% cap eta to -pi/2 to pi/2
eta = min(eta, pi/2);
eta = max(eta, -pi/2);

lacc = 2*(groundSpeed^2)/L1*sin(eta);

rollSP = atan(lacc/9.81);

== matlab function eVTOL_System/Flight Controller/Autopilot/Fixed Wing Controller/Fixed Wing Controller Tuning/Attitude Controller/Pitch Roll Controller/Turn Coordinator/MATLAB Function ==
  data: rollSP input; rSP output; pitchSP input; airSpeed input
function rSP = fcn(rollSP, pitchSP, airSpeed)
    yawRateSP = tan(rollSP)*9.81/airSpeed;
    rSP = yawRateSP*cos(pitchSP)*cos(rollSP);
end

== matlab function eVTOL_System/Flight Controller/Autopilot/Multicopter Controller/Horizontal Position Control/XY Controller/Yaw Correction ==
  data: xcmd input; ucmd output; ycmd input; yaw input; vcmd output
function [ucmd,vcmd] = fcn(xcmd,ycmd,yaw)
%xcmd acceleration in NED X direction
ucmd=xcmd*cos(yaw)+ycmd*sin(yaw);
vcmd=-xcmd*sin(yaw)+ycmd*cos(yaw);
end

== matlab function eVTOL_System/Flight Controller/Guidance Test Bench/ControlType/Guidance Testbench/Guidance Logic/Guidance Stateflow/Guidance Mode Selector/GuidanceLogic.BackTransition.BackTransition/MATLAB Function ==
  data: Vb input; tilt input; flag output
function flag = fcn(Vb,tilt)
tiltConditionMet=abs(tilt)<1e-1;
velocityConditionMet=abs(norm([Vb(1) 0 0]))<4;

flag=tiltConditionMet&velocityConditionMet;
end
